simulink model "stimlib"  (Simulink 7.0)
settings: Solver=ode45  SolverMode=SingleTasking  StartTime=0.0  StopTime=999999  MaxStep=10  RelTol=1e-3  AbsTol=1e-3
undefined symbols (not defined in the file or in its folder): sigbuilder_block
settings Model: Creator=jacobs  LastModifiedBy=lfd  ExtModeAutoUpdateStatusClock=off
settings DataIOCC: LimitDataPoints=off  SaveOutput=off  SaveTime=off
settings OptimizationCC: BlockReduction=off  BooleanDataType=off
settings DebuggingCC: SaveWithParameterizedLinksMsg=none  SignalResolutionControl=TryResolveAllWithWarning  SolverPrmCheckMsg=none  MultiTaskDSMMsg=warning  MultiTaskCondExecSysMsg=none  StrictBusMsg=None
settings HardwareCC: TargetUnknown=on
settings RTWCC: IncludeERTFirstTime=on
settings GRTTargetCC: TargetFcnLib=ansi_tfl_tmw.mat  ModelReferenceCompliant=off  CompOptLevelCompliant=off  MatFileLogging=off

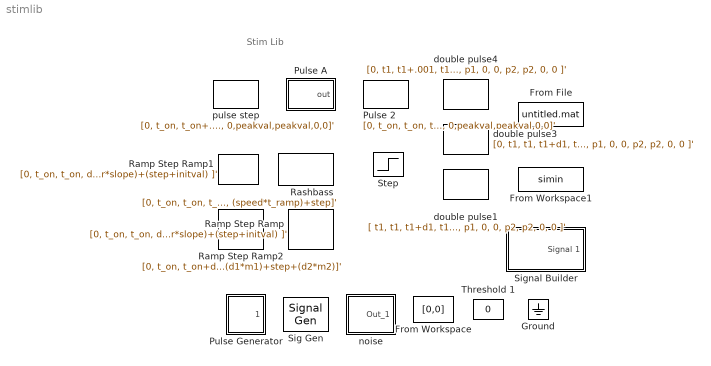
== system stimlib ==
  note: Stim Lib
  From Workspace : FromWorkspace  VariableName=[0,0]  SampleTime=.001
  From Workspace1 : FromWorkspace  VariableName=simin  SampleTime=0
  From File : FromFile  SampleTime=0
  Ground : Ground
  Pulse Generator : Subsystem  mask(Pulse Generator){@1=.5, @2=.04, @3=2, @4=.1}
      mask prompts: @1 "Pulse period (secs):"; @2 "Pulse width:"; @3 "Pulse height:"; @4 "Pulse start time:"
      mask help: Pulse Generator.
      mask init:
      | Ts=@1; du=@2; ht=@3; stt=@4; ini=ones(length(ht),1); st1=rem(stt,Ts); st2=rem(stt+du,Ts);if(Ts<=1.2*du),ini=zeros(length(ht),1);end;
      mask Help: Pulse generator which ensures pulse\ntransitions are hit. Provides a vector of pulses when the height is entered as a vector.\nUnmask to see how it works.
      mask Display: plot(0,0,100,100,[90,75,75,60,60,35,35,20,20,10],[20,20,80,80,20,20,80,80,20,20])
  Pulse 2 : FromWorkspace  VariableName=[0, t_on, t_on, t_on+dur,t_on+dur 5; 0, 0,peakval,peakval,0,0]'  mask{@1=1, @2=0, @3=1}
      mask prompts: @1 "Peak value"; @2 "Time of step"; @3 "Step duration"
      mask help: Pulse
      mask init:
      | peakval = @1; t_on = @2; dur = @3;
      mask Display: disp('Pulse2')
  Pulse A : Subsystem  mask{@1=0, @2=1, @3=2}
      mask prompts: @1 "Time of onset:"; @2 "Peak value:"; @3 "Time of offset:"
      mask help: Single Pulse
      mask init:
      | onsetTime = @1; peak = @2; offsetTime = @3;
      mask Display: disp('pulse')
  Ramp Step Ramp : FromWorkspace  VariableName=[0, t_on, t_on, dur; initval, (t_on*slope)+initval, (t_on*slope)+(step+initval), (dur*slope)+(step+initval) ]'  mask{initval=-5, t_on=1, step=5, dur=2, slope=5}
      mask prompts: initval "Initial value"; t_on "Time of step"; step "Size of step"; dur "Ramp duration"; slope "Ramp slope"
      mask help: Ramp Step Ramp
      mask Display: disp('Ramp\nStep\nRamp2')
  Ramp Step Ramp1 : FromWorkspace  VariableName=[0, t_on, t_on, dur+t_on dur+t_on; initval, initval, initval+step, (dur*slope)+(step+initval), (dur*slope)+(step+initval) ]'  mask{initval=0, t_on=1, step=5, dur=2, slope=5}
      mask prompts: initval "Initial value"; t_on "Time of step"; step "Size of step"; dur "Ramp duration"; slope "Ramp slope"
      mask help: Ramp Step Ramp
      mask Display: disp('Step\nRamp')
  Ramp Step Ramp2 : FromWorkspace  VariableName=[0, t_on, t_on+d1, t_on+d1, t_on+d1+d2, 10000; vi, vi, vi+(d1*m1), (vi+step)+(d1*m1), (vi+step)+(d1*m1)+(d2*m2), vi+(d1*m1)+step+(d2*m2)]'  mask{vi=-5, t_on=1, d1=2, m1=5, step=-10, d2=2, m2=10}
      mask prompts: vi "Initial value"; t_on "Time of first ramp"; d1 "First Ramp duration"; m1 "First Ramp slope"; step "Size of step"; d2 "Second Ramp duration"; m2 "Second Ramp slope"
      mask help: Ramp Step Ramp
      mask Display: disp('Ramp\nStep\nRamp')
  Rashbass : FromWorkspace  VariableName=[0, t_on, t_on, t_ramp+t_on; initval, initval, step, (speed*t_ramp)+step]'  mask{@1=0, @2=0.5, @3=-2, @4=10, @5=5}
      mask prompts: @1 "Initial value"; @2 "Time of step"; @3 "Size of step"; @4 "Ramp duration"; @5 "Ramp slope"
      mask help: Rashbass
      mask init:
      | initval = @1; t_on = @2; step = @3; t_ramp = @4; speed = @5;
      mask Display: disp('Rashbass')
  Sig Gen : SignalGenerator  WaveForm=square  Amplitude=1.000000  Frequency=10.000000  Units=rad/sec
  Signal Builder : Subsystem  Tag=STV Subsys  LoadFcn=sigbuilder_block('load');  StartFcn=sigbuilder_block('start');  StopFcn=sigbuilder_block('stop');  ClipboardFcn=sigbuilder_block('clipboard');  mask(Sigbuilder block){}
      mask help: Sigbuilder GUI
      mask init:
      | if ~strcmp(get_param(bdroot(gcbh),'SimulationStatus'),'stopped') tuvar = sigbuilder_block('maskInit'); end
      settings: CopyFcn=sigbuilder_block('copy');  DeleteFcn=sigbuilder_block('delete');  ModelCloseFcn=sigbuilder_block('modelClose');  PreSaveFcn=sigbuilder_block('preSave');  NameChangeFcn=sigbuilder_block('namechange');  OpenFcn=sigbuilder_block('open',[437.6 199.2 550.4 400 ]);  CloseFcn=sigbuilder_block('close');
      mask Display: plot(0,0,100,100,[10,10,40,40,10],[80,20,20,80,80],[40,10],[50,50], [40,27,10],[65,72,56],[40,25,25,10],[28,28,43,43]);
  Step : Step  Time=.1  After=4
  Threshold 1 : Constant  Value=0  OutDataType=sfix(16)  OutScaling=2^0
  double pulse1 : FromWorkspace  VariableName=[ t1, t1, t1+d1, t1+d1, t1+d1+ipd, t1+d1+ipd, t1+d1+ipd+d2, t1+d1+ipd+d2, 10000; 0, p1, p1, 0, 0, p2, p2, 0, 0 ]'  mask{@1=goal, @2=0.01, @3=stoptime, @4=0, @5=0, @6=0}
      mask prompts: @1 "Pulse 1 Magnitude"; @2 "Time of Pulse 1 Onset"; @3 "Pulse 1 Duration"; @4 "Interpulse Delay"; @5 "Pulse 2 Magnitude"; @6 "Pulse 2 Duration"
      mask help: Double Pulse
      mask init:
      | p1=@1; t1=@2; d1=@3; ipd=@4; p2=@5; d2=@6;
      mask Display: disp('Double\nPulse3')
  double pulse3 : FromWorkspace  VariableName=[0, t1, t1, t1+d1, t1+d1, t1+d1+ipd, t1+d1+ipd, t1+d1+ipd+d2, t1+d1+ipd+d2, 10000; 0, 0, p1, p1, 0, 0, p2, p2, 0, 0 ]'  mask{@1=goal, @2=0, @3=stoptime, @4=0, @5=0, @6=0}
      mask prompts: @1 "Pulse 1 Magnitude"; @2 "Time of Pulse 1 Onset"; @3 "Pulse 1 Duration"; @4 "Interpulse Delay"; @5 "Pulse 2 Magnitude"; @6 "Pulse 2 Duration"
      mask help: Double Pulse
      mask init:
      | p1=@1; t1=@2; d1=@3; ipd=@4; p2=@5; d2=@6;
      mask Display: disp('Double\nPulse2')
  double pulse4 : FromWorkspace  VariableName=[0, t1, t1+.001, t1+d1, t1+d1+.001, t1+d1+.001+ipd, t1+d1+.001+ipd, t1+d1+.001+ipd+d2, t1+d1+.001+ipd+d2, 10000; 0, 0, p1, p1, 0, 0, p2, p2, 0, 0 ]'  mask{@1=goal, @2=0, @3=stoptime, @4=0, @5=0, @6=0}
      mask prompts: @1 "Pulse 1 Magnitude"; @2 "Time of Pulse 1 Onset"; @3 "Pulse 1 Duration"; @4 "Interpulse Delay"; @5 "Pulse 2 Magnitude"; @6 "Pulse 2 Duration"
      mask help: Double Pulse
      mask init:
      | p1=@1; t1=@2; d1=@3; ipd=@4; p2=@5; d2=@6;
      mask Display: disp('Double\nPulse')
  noise : Subsystem  mask(Continuous White Noise.){@1=[0.0001], @2=0.001, @3=[23341]}
      mask prompts: @1 "Noise Power:"; @2 "Sample Time:"; @3 "Seed"
      mask help:
      | White noise for continuous (s-domain) systems.
      | Band-limited using zero-order-hold.
      mask init:
      | Cov = @1; Ts = @2; seed = @3; r = rand(1,12); r2 = [r(1),r;r,r(12)]; t =[1:13;1:13];
      mask Help: Implemented using white noise into Zero-Order Hold block. The seed and power can be vectors of the same length to produce a vector of white noise sources. For faster simulation, set sample time to the highest value possible but in accordance with the fastest dynamics of system.
      mask Display: plot(t(:),r2(:))
  pulse step : FromWorkspace  VariableName=[0, t_on, t_on+.001, t_on+dur,t_on+dur+.001 500000; 0, 0,peakval,peakval,0,0]'  mask{@1=5, @2=0, @3=.02}
      mask prompts: @1 "Peak value"; @2 "Time of step"; @3 "Step duration"
      mask help: Pulse
      mask init:
      | peakval = @1; t_on = @2; dur = @3;
      mask Display: disp('Pulse')

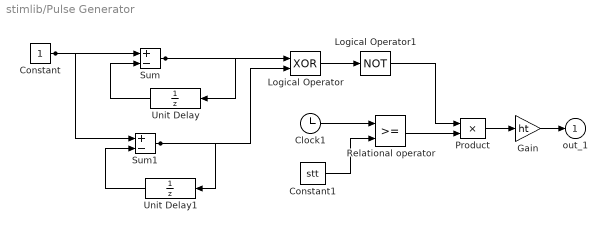
== system stimlib/Pulse Generator ==
  Clock1 : Clock
      settings: Decimation=10
  Constant : Constant  OutDataType=sfix(16)  OutScaling=2^0
  Constant1 : Constant  Value=stt  OutDataType=sfix(16)  OutScaling=2^0
  Gain : Gain  Gain=ht  ParameterDataType=sfix(16)  ParameterScaling=2^0  OutDataType=sfix(16)  OutScaling=2^0  SaturateOnIntegerOverflow=on
  Logical Operator : Logic  Operator=XOR
  Logical Operator1 : Logic  Operator=NOT  Inputs=1
  Product : Product  OutDataType=sfix(16)  OutScaling=2^0  SaturateOnIntegerOverflow=on  RndMeth=Zero  InputSameDT=on
  Relational operator : RelationalOperator  InputSameDT=on
  Sum : Sum  Inputs=+-  OutDataType=sfix(16)  OutScaling=2^0  SaturateOnIntegerOverflow=on  InputSameDT=on
  Sum1 : Sum  Inputs=+-  OutDataType=sfix(16)  OutScaling=2^0  SaturateOnIntegerOverflow=on  InputSameDT=on
  Unit Delay : UnitDelay  Orientation=left  SampleTime=[Ts,st1]
  Unit Delay1 : UnitDelay  Orientation=left  X0=ini  SampleTime=[Ts,st2]
  out_1 : Outport  OutDataType=sfix(16)  OutScaling=2^0  InitialOutput=0
  wires:
  Sum1/1 -> Logical Operator/2, Unit Delay1/1
  Sum/1 -> Logical Operator/1, Unit Delay/1
  Constant/1 -> Sum1/1, Sum/1
  Unit Delay1/1 -> Sum1/2
  Unit Delay/1 -> Sum/2
  Clock1/1 -> Relational operator/1
  Relational operator/1 -> Product/2
  Product/1 -> Gain/1
  Gain/1 -> out_1/1
  Constant1/1 -> Relational operator/2
  Logical Operator/1 -> Logical Operator1/1
  Logical Operator1/1 -> Product/1

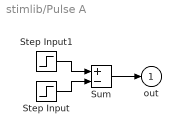
== system stimlib/Pulse A ==
  Step Input : Step  Time=offsetTime  After=peak
  Step Input1 : Step  Time=onsetTime  After=peak
  Sum : Sum  Inputs=+-  OutDataType=sfix(16)  OutScaling=2^0  SaturateOnIntegerOverflow=on  InputSameDT=on
  out : Outport  OutDataType=sfix(16)  OutScaling=2^0  InitialOutput=0
  wires:
  Sum/1 -> out/1
  Step Input1/1 -> Sum/1
  Step Input/1 -> Sum/2

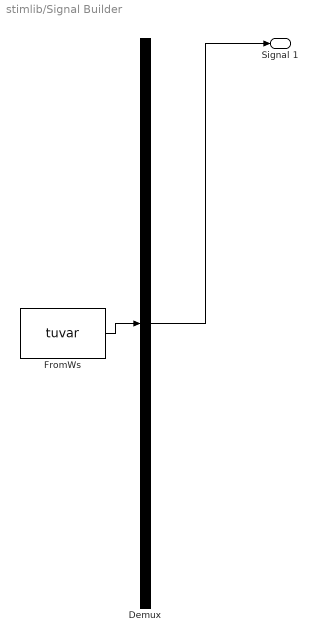
== system stimlib/Signal Builder ==
  Demux : Demux  Tag=STV Demux  Outputs=1
  FromWs : FromWorkspace  Tag=STV FromWs  VariableName=tuvar  SampleTime=0  SigBuilderData=DataTag0  VnvData=DataTag1
      SigBuilderData=|
      | channels.label = 'Signal 1'
      | channels.allXData = {[0 4 4 6 6 10]}
      | channels.allYData = {[0 0 1 1 0 0]}
      | common.afterFinalStr = 'Extrapolate'
      | common.sampleTime = 0
      | dataSet.timeRange = [0 10]
      | dataSet.name = 'Group 1'
  Signal 1 : Outport  Tag=STV Outport  OutDataType=sfix(16)  OutScaling=2^0
  wires:
  Demux/1 -> Signal 1/1
  FromWs/1 -> Demux/1

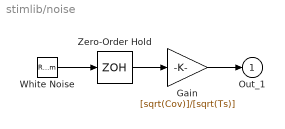
== system stimlib/noise ==
  Gain : Gain  Gain=[sqrt(Cov)]/[sqrt(Ts)]  ParameterDataType=sfix(16)  ParameterScaling=2^0  OutDataType=sfix(16)  OutScaling=2^0  SaturateOnIntegerOverflow=on
  White Noise : RandomNumber  Seed=seed  SampleTime=.001
  Zero-Order Hold : ZeroOrderHold  SampleTime=Ts
  Out_1 : Outport  OutDataType=sfix(16)  OutScaling=2^0  InitialOutput=0
  wires:
  White Noise/1 -> Zero-Order Hold/1
  Gain/1 -> Out_1/1
  Zero-Order Hold/1 -> Gain/1
